simulink model "gm_model_biquad_wfa_interface_modified"  (R2020b)
settings: Solver=FixedStepDiscrete  StartTime=0.0  StopTime=inf  RelTol=1e-3  EnableMultiTasking=on
values from neighbouring files (symbols this model uses):
  in_cos = 2*cos(2*pi*k/N)    [compute_constants.m]    (also in signat_to_test_generate.m = -2*cos(2*pi*k/N))
  Ts = 1e-3    (= 0.001)    [compute_constants.m]    (also in signat_to_test_generate.m)
  Wkn = -exp(-j*2*pi*k/N)    [compute_constants.m]    (also in signat_to_test_generate.m)
undefined symbols (not defined in the file or in its folder): AXI4, ip, Lite
libraries: axi_iio_lib x2, axiinterfacelib x2
settings Model: Creator=pablo  LastModifiedBy=pablo
settings SolverCC: ConcurrentTasks=on  PositivePriorityOrder=on
settings OptimizationCC: EnhancedBackFolding=on  PassReuseOutputArgsAs=Individual arguments  ZeroExternalMemoryAtStartup=off  ZeroInternalMemoryAtStartup=off  MaxStackSize=64  OptimizeBlockOrder=speed  DifferentSizesBufferReuse=on  OptimizationCustomize=off  EfficientTunableParamExpr=on
settings DebuggingCC: ParameterTunabilityLossMsg=error
settings HardwareCC: ProdBitPerPointer=32  ProdBitPerSizeT=32  ProdBitPerPtrDiffT=32  ProdLargestAtomicInteger=Long  ProdLargestAtomicFloat=Double  ProdWordSize=32  ProdLongLongMode=on  ProdHWDeviceType=ARM Compatible->ARM Cortex  TargetBitPerPointer=64  TargetBitPerSizeT=64  TargetBitPerPtrDiffT=64  TargetLargestAtomicFloat=Float  TargetIntDivRoundTo=Zero  TargetEndianess=LittleEndian  TargetWordSize=64  TargetHWDeviceType=Intel->x86-64 (Windows64)
settings SFSimCC: MATLABDynamicMemAlloc=off
settings RTWCC: Description=Embedded Coder  SystemTargetFile=ert.tlc  HardwareBoard=Xilinx Zynq-7000 based board  TLCOptions="-aInlineSetEventsForThisBaseRateFcn=TLC_FALSE -aSuppressMultiTaskScheduler=TLC_FALSE  -aRateBasedStepFcn=0"  TemplateMakefile=ert_default_tmf  Toolchain=Linaro AArch32 Linux v6.3.1
settings CodeAppCC: ForceParamTrailComments=on  IgnoreCustomStorageClasses=off  OperatorAnnotations=on  SimulinkDataObjDesc=on  SFDataObjDesc=on  InsertBlockDesc=on

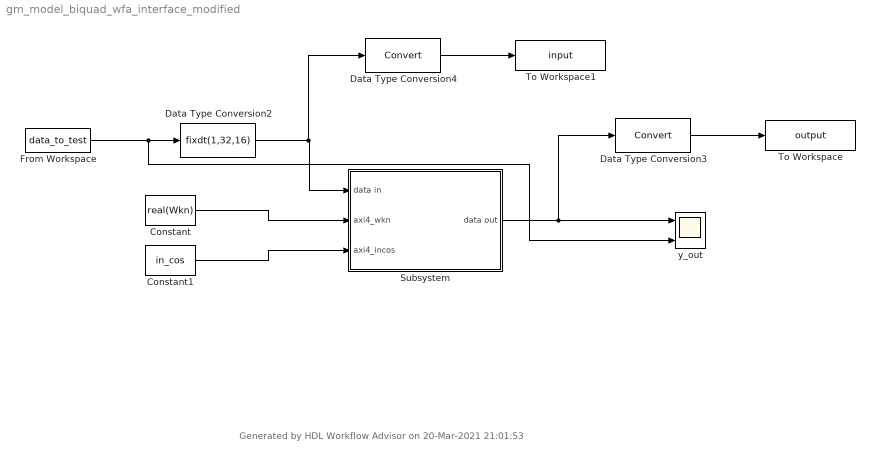
== system gm_model_biquad_wfa_interface_modified ==
  note: Generated by HDL Workflow Advisor on 20-Mar-2021 21:01:53
  Constant : Constant  Value=real(Wkn)  OutDataTypeStr=fixdt(1,32,16)  SampleTime=Ts
  Constant1 : Constant  Value=in_cos  OutDataTypeStr=fixdt(1,32,16)  SampleTime=Ts
  Data Type Conversion2 : DataTypeConversion  OutDataTypeStr=fixdt(1,32,16)
  Data Type Conversion3 : DataTypeConversion
  Data Type Conversion4 : DataTypeConversion
  From Workspace : FromWorkspace  VariableName=data_to_test  SampleTime=Ts  Interpolate=off  OutputAfterFinalValue=Cyclic repetition
  Subsystem : Subsystem
  To Workspace : ToWorkspace  VariableName=output  SaveFormat=Structure  SampleTime=Ts
  To Workspace1 : ToWorkspace  VariableName=input  SaveFormat=Structure  SampleTime=Ts
  y_out : Scope  NumInputPorts=2
  wires:
  Constant/1 -> Subsystem/2(axi4_wkn)
  Constant1/1 -> Subsystem/3(axi4_incos)
  From Workspace/1 -> y_out/2, Data Type Conversion2/1
  Subsystem/1(data out) -> y_out/1, Data Type Conversion3/1
  Data Type Conversion3/1 -> To Workspace/1
  Data Type Conversion4/1 -> To Workspace1/1
  Data Type Conversion2/1 -> Subsystem/1(data in), Data Type Conversion4/1

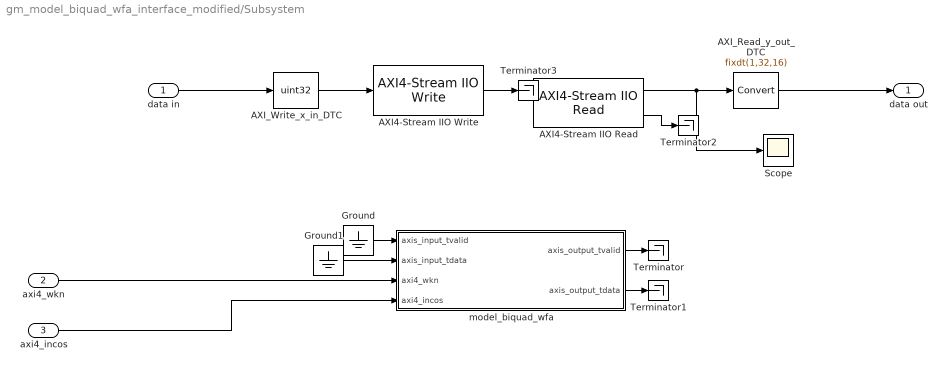
== system gm_model_biquad_wfa_interface_modified/Subsystem ==
  data in : Inport
  axi4_wkn : Inport  Port=2
  axi4_incos : Inport  Port=3
  AXI4-Stream IIO Read : axi_iio_lib/AXI4-Stream IIO Read  devName=mwipcore0:s2mm0  SamplesPerFrame=32  dataTypeStr=uint32  tLastMode=auto  resetTlastMode=prebuffer  SampleTime=Ts  DataTimeout=10  uri=ip:10.0.0.200  enIO=off
      settings: SourceProductBaseCode=HDL_ALTERA_SOC,INTEL_FPGA_SOC,XILINX_FPGA_SOC,INTEL_BLOCKSET,USRPEMBED,XILINX_BLOCKSET,HCZYNQ7000,ECZYNQ7000,XILINXZYNQ,VP_VISION_ZYNQ
  AXI4-Stream IIO Write : axi_iio_lib/AXI4-Stream IIO Write  Priority=1  devName=mwipcore0:mm2s0  DataTimeout=0  uri=ip:10.0.0.200  enIO=off
      settings: SourceProductBaseCode=HDL_ALTERA_SOC,INTEL_FPGA_SOC,XILINX_FPGA_SOC,INTEL_BLOCKSET,USRPEMBED,XILINX_BLOCKSET,HCZYNQ7000,ECZYNQ7000,XILINXZYNQ,VP_VISION_ZYNQ
  AXI_Read_y_out_DTC : DataTypeConversion  OutDataTypeStr=fixdt(1,32,16)  ConvertRealWorld=Stored Integer (SI)
  AXI_Write_x_in_DTC : DataTypeConversion  OutDataTypeStr=uint32  ConvertRealWorld=Stored Integer (SI)
  Ground : Ground
  Ground1 : Ground
  Scope : Scope
  Terminator{,1..3} (4 alike) : Terminator
  model_biquad_wfa : Subsystem  TreatAsAtomicUnit=on  mask(AXI4-Lite/AXI4 Interface){}
      mask help:
      | This is an automatically generated subsystem block.
      | This contains the AXI interface blocks that communicate with the axis_goertzel_ip IPCore generated from model_biquad_wfa subsystem.
      mask Display: disp(sprintf('Xilinx Zynq \nAXI Interface'));
  data out : Outport
  wires:
  data in/1 -> AXI_Write_x_in_DTC/1
  model_biquad_wfa/1(axis_output_tvalid) -> Terminator/1
  AXI_Write_x_in_DTC/1 -> AXI4-Stream IIO Write/1
  Ground1/1 -> model_biquad_wfa/2(axis_input_tdata)
  model_biquad_wfa/2(axis_output_tdata) -> Terminator1/1
  axi4_wkn/1 -> model_biquad_wfa/3(axi4_wkn)
  axi4_incos/1 -> model_biquad_wfa/4(axi4_incos)
  Ground/1 -> model_biquad_wfa/1(axis_input_tvalid)
  AXI4-Stream IIO Read/1 -> Scope/1, AXI_Read_y_out_DTC/1
  AXI4-Stream IIO Read/2 -> Terminator2/1
  AXI_Read_y_out_DTC/1 -> data out/1
  AXI4-Stream IIO Write/1 -> Terminator3/1

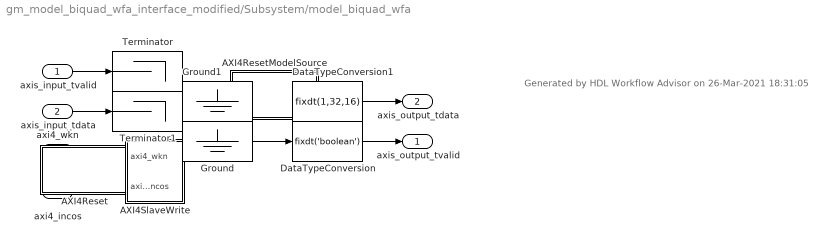
== system gm_model_biquad_wfa_interface_modified/Subsystem/model_biquad_wfa ==
  note: Generated by HDL Workflow Advisor on 26-Mar-2021 18:31:05
  axis_input_tvalid : Inport
  axis_input_tdata : Inport  Port=2
  axi4_wkn : Inport  Port=3
  axi4_incos : Inport  Port=4
  AXI4Reset : Subsystem  mask(System Start){ShowInLibBrowser=0}
      mask prompts: ShowInLibBrowser "Simulink:masks:CustCodeMaskParam1_MP"
      settings: CopyFcn=cccopyfcn(gcb)  OpenFcn=ccopenfcn('System Start Function')
      mask Help: eval('feval(''rtwprivate'',''rtwhelpview'',''rtw_sys_start_block'')');
      mask Display: disp('System\nStart');
  AXI4ResetModelSource : Subsystem  mask(Model Source){ShowInLibBrowser=0}
      mask prompts: ShowInLibBrowser "Simulink:masks:CustCodeMaskParam1_MP"
      settings: CopyFcn=cccopyfcn(gcb)  OpenFcn=ccopenfcn('Model Source')
      mask Help: eval('feval(''rtwprivate'',''rtwhelpview'',''rtw_model_source_block'')');
      mask Display: disp('Model\nSource');
  AXI4SlaveWrite : Subsystem  Priority=1
  DataTypeConversion : DataTypeConversion  OutDataTypeStr=fixdt('boolean')  ConvertRealWorld=Stored Integer (SI)
  DataTypeConversion1 : DataTypeConversion  OutDataTypeStr=fixdt(1,32,16)  ConvertRealWorld=Stored Integer (SI)
  Ground : Ground
  Ground1 : Ground
  Terminator : Terminator
  Terminator1 : Terminator
  axis_output_tvalid : Outport
  axis_output_tdata : Outport  Port=2
  wires:
  axi4_wkn/1 -> AXI4SlaveWrite/1(axi4_wkn)
  axi4_incos/1 -> AXI4SlaveWrite/2(axi4_incos)
  axis_input_tvalid/1 -> Terminator/1
  axis_input_tdata/1 -> Terminator1/1
  DataTypeConversion/1 -> axis_output_tvalid/1
  Ground/1 -> DataTypeConversion/1
  DataTypeConversion1/1 -> axis_output_tdata/1
  Ground1/1 -> DataTypeConversion1/1

== system gm_model_biquad_wfa_interface_modified/Subsystem/model_biquad_wfa/AXI4Reset ==

== system gm_model_biquad_wfa_interface_modified/Subsystem/model_biquad_wfa/AXI4ResetModelSource ==

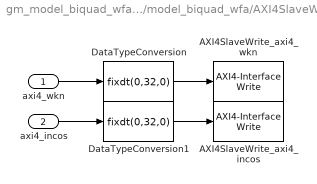
== system gm_model_biquad_wfa_interface_modified/Subsystem/model_biquad_wfa/AXI4SlaveWrite ==
  axi4_wkn : Inport
  axi4_incos : Inport  Port=2
  AXI4SlaveWrite_axi4_incos : axiinterfacelib/AXI4-Interface Write  Priority=2  AXIInterfaceType=AXI4-Lite  DeviceName=/dev/mwipcore  RegisterOffset=hex2dec('100')  blockPlatform=ZYNQ  SimulateUsing=Interpreted execution
      settings: SourceProductBaseCode=ECZYNQ7000
  AXI4SlaveWrite_axi4_wkn : axiinterfacelib/AXI4-Interface Write  Priority=1  AXIInterfaceType=AXI4-Lite  DeviceName=/dev/mwipcore  RegisterOffset=hex2dec('104')  blockPlatform=ZYNQ  SimulateUsing=Interpreted execution
      settings: SourceProductBaseCode=ECZYNQ7000
  DataTypeConversion : DataTypeConversion  OutDataTypeStr=fixdt(0,32,0)  ConvertRealWorld=Stored Integer (SI)
  DataTypeConversion1 : DataTypeConversion  OutDataTypeStr=fixdt(0,32,0)  ConvertRealWorld=Stored Integer (SI)
  wires:
  DataTypeConversion/1 -> AXI4SlaveWrite_axi4_wkn/1
  axi4_wkn/1 -> DataTypeConversion/1
  axi4_incos/1 -> DataTypeConversion1/1
  DataTypeConversion1/1 -> AXI4SlaveWrite_axi4_incos/1
